simulink model "Pendulo"  (R2021a)
settings: Solver=VariableStepAuto  StartTime=0.0  StopTime=10.0  RelTol=1e-3
values from neighbouring files (symbols this model uses):
  kTc = 1/(m*l*l)    (= 1)    [script.m]
  w0 = sqrt(g/l)    [script.m]
settings Model: Creator=taffarel55  LastModifiedBy=taffarel55

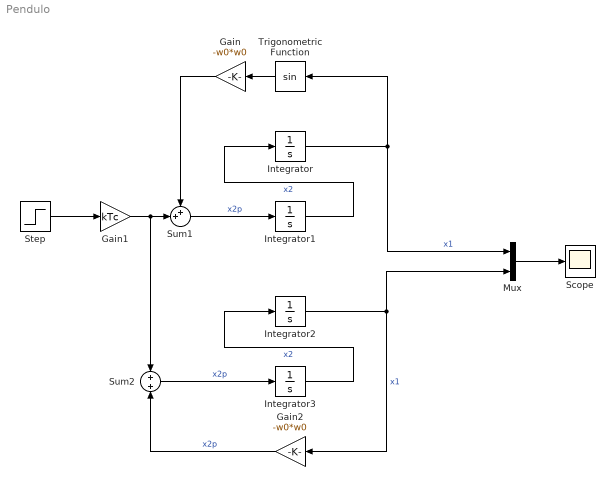
== system Pendulo ==
  Gain : Gain  Gain=-w0*w0
  Gain1 : Gain  Gain=kTc
  Gain2 : Gain  Gain=-w0*w0
  Integrator{,1..3} (4 alike) : Integrator
  Mux : Mux  Inputs=2
  Scope : Scope
  Step : Step  After=5  SampleTime=0
  Sum1 : Sum  Inputs=++|
  Sum2 : Sum  Inputs=+|+
  Trigonometric Function : Trigonometry
  wires:
  Integrator/1 -> Mux/1, Trigonometric Function/1  "x1"
  Sum1/1 -> Integrator1/1  "x2p"
  Integrator1/1 -> Integrator/1  "x2"
  Trigonometric Function/1 -> Gain/1
  Step/1 -> Gain1/1
  Gain1/1 -> Sum2/1, Sum1/2
  Gain/1 -> Sum1/1
  Integrator3/1 -> Integrator2/1  "x2"
  Integrator2/1 -> Gain2/1, Mux/2  "x1"
  Gain2/1 -> Sum2/2  "x2p"
  Sum2/1 -> Integrator3/1  "x2p"
  Mux/1 -> Scope/1
